simulink model "EMPlanner_cs_old"  (R2020a)
settings: Solver=ode5  StartTime=0.0  StopTime=55  FixedStep=1/1000  RelTol=1e-3
PreLoadFcn:
  | mbxruntime.callbacks.PreLoadFcn(bdroot);
PostLoadFcn:
  | mbxruntime.callbacks.PostLoadFcn(bdroot);
InitFcn:
  | mbxruntime.callbacks.InitFcn(bdroot);
StartFcn:
  | mbxruntime.callbacks.StartFcn(bdroot);
StopFcn:
  | mbxruntime.callbacks.StopFcn(bdroot);
model workspace: external: MAT-File .\EMPlanner_cs_hws.mat (data not in the file)
values from neighbouring files (symbols this model uses):
  c_factor = 43.75    [emplanner_init.m]
  cf = -175016    [emplanner_init.m]
  cr = -130634    [emplanner_init.m]
  KD_PID_distance = 0.0    (= 0)    [emplanner_init.m]
  KD_PID_speed = 0    [emplanner_init.m]
  KI_PID_distance = 0.0    (= 0)    [emplanner_init.m]
  KI_PID_speed = 0    [emplanner_init.m]
  KP_PID_distance = 0.5    [emplanner_init.m]
  KP_PID_speed = 1.8    [emplanner_init.m]
  la = 1.265    [emplanner_init.m]
  lb = 2.947-1.265    (= 1.682)    [emplanner_init.m]
  LQR_K1 = k(:,1)'    [emplanner_init.m]
  LQR_K2 = k(:,2)'    [emplanner_init.m]
  LQR_K3 = k(:,3)'    [emplanner_init.m]
  LQR_K4 = k(:,4)'    [emplanner_init.m]
  m = 2020    [emplanner_init.m]
  path_x = [7.7742 8.77358225507 9.77170536558 10.7685522493 11.7641171228 12.7583983581 13.7513958557 14.7431100776 15.7335416918 16.7226914411 17.7105600952 18.6971484329 ... (551 elements, 551x1)]    [test_path.mat]
  path_y = [-207.8202 -207.82020006 -207.820200616 -207.820202023 -207.82020429 -207.820207237 -207.820210603 -207.820214131 -207.82021762 -207.820220941 -207.820224011 -207.820226778 ... (551 elements, 551x1)]    [test_path.mat]
  rack_displacement = [-39.14 , -37.2 , -35.29 , -33.43 , -31.6 , -29.81 , -28.06 , -26.34 , -24.66 ,      -23.01 , -21.38 , -19.79 , -18.23 , -16.69 , -15.18 , -13.7 , -12.23 , -10.8 , -9.38 , -7.98 ,     -6.61 , -5.25 , -3.91 , -2.59 , -1.29 , 0 , 1.27 , 2.54 , 3.78 , 5.02 , 6.24 , 7.46 , 8.66 ,      9.86 , 11.05 , 12.24 , 13.41 , 14.59 , 15.76 , 16.92 , 18.09 , 19.25 , 20.42 , 21.59 , 22.76 ,      23.93 , 25.11 , 26 ...(+26 chars)    [emplanner_init.m]
  right_wheel_ground = [-70 ,-67.2 , -64.4 , -61.6 , -58.8 , -56 , -53.2 , -50.4 , -47.6 , -44.8 , -42 ,      -39.2 , -36.4 , -33.6 , -30.8 , -28 , -25.2 , -22.4 , -19.6 , -16.8 , -14 , -11.2 , -8.4 , -5.6 ,      -2.8 , 0 , 2.8 , 5.6 , 8.4 , 11.2 , 14 , 16.8 , 19.6 , 22.4 , 25.2 , 28 , 30.8 , 33.6 , 36.4 ,      39.2 , 42 , 44.8 , 47.6 , 50.4 , 53.2 , 56 , 58.8 , 61.6 , 64.4 , 67.2 , 70 ]    [emplanner_init.m]
  vx_break_point = zeros(1,5000)    [emplanner_init.m]
undefined symbols (not defined in the file or in its folder): aubr, DiscIntNeverNeededParam, tablebr, vubr, warningInitialVelocity, x0
libraries: simulink x19, PreScanSimulinkLibrary x10, simulink_extras x5, Solver_SF x1
(part 8 of 8)

== matlab function EMPlanner_cs_old/Audi_A8_Sedan_1/decision&planning module/EM Planner/Frenet2Cartesian ==
  data: s_set_fcs input; x_set_gcs output; l_set_fcs input; dl_set_fcs input; ddl_set_fcs input; path_x_set_gcs input; path_y_set_gcs input; path_heading_set_gcs input; path_kappa_set_gcs input; matchPoint_index_s_set_fcs input; y_set_gcs output; heading_set_gcs output; kappa_set_gcs output
function [x_set_gcs,y_set_gcs,heading_set_gcs,kappa_set_gcs] = fcn(s_set_fcs,l_set_fcs,dl_set_fcs,ddl_set_fcs,...
    path_x_set_gcs,path_y_set_gcs,path_heading_set_gcs,path_kappa_set_gcs,matchPoint_index_s_set_fcs)
% 该函数将批量将(s,l) 转化成 (x,y)
% s_set_fcs,l_set_fcs,dl_set_fcs,ddl_set_fcs 转换点 自然坐标系信息
% path_x_set_gcs,path_y_set_gcs,path_heading_set_gcs,path_kappa_set_gcs 给定路径采样点信息
% matchPoint_index_s_set_fcs 给定路径采样点s坐标集合
% 假设最多有181个点需要转换
n = 181;
% 输出初始化
x_set_gcs = ones(n,1)*nan; y_set_gcs = ones(n,1)*nan; heading_set_gcs = ones(n,1)*nan; kappa_set_gcs = ones(n,1)*nan;
for i = 1:length(s_set_fcs)
    if isnan(s_set_fcs(i))
        break;
    end
    % 求出该点在给定路径采样点上 投影点的信息
    [proj_point_x_gcs,proj_point_y_gcs,proj_point_heading_gcs,proj_point_kappa_gcs] = ...
                CalProjPointInfoFromFrenet(s_set_fcs(i),path_x_set_gcs,path_y_set_gcs,path_heading_set_gcs,...
                                                path_kappa_set_gcs,matchPoint_index_s_set_fcs);
    x_set_gcs(i) = proj_point_x_gcs - l_set_fcs(i) * sin(proj_point_heading_gcs);
    y_set_gcs(i) = proj_point_y_gcs + l_set_fcs(i) * cos(proj_point_heading_gcs);
    heading_set_gcs(i) = proj_point_heading_gcs + atan(dl_set_fcs(i)/(1-proj_point_kappa_gcs*l_set_fcs(i)));
    k1 = ddl_set_fcs(i) + proj_point_kappa_gcs * dl_set_fcs(i) * tan(heading_set_gcs(i)-proj_point_heading_gcs);
    k2 = (cos(heading_set_gcs(i)-proj_point_heading_gcs))^2 / (1 - proj_point_kappa_gcs*l_set_fcs(i));
    k3 = cos(heading_set_gcs(i)-proj_point_heading_gcs) / (1 - proj_point_kappa_gcs*l_set_fcs(i));
    kappa_set_gcs(i) = (k1 * k2 + proj_point_kappa_gcs) * k3;
end
end

== matlab function EMPlanner_cs_old/Audi_A8_Sedan_1/decision&planning module/EM Planner/path and speed merge ==
  data: s input; trajectory_x output; s_dot input; s_dot2 input; relative_time input; current_time input; path_s input; trajectory_x_init input; trajectory_y_init input; trajectory_heading_init input; trajectory_kappa_init input; trajectory_y output; trajectory_heading output; trajectory_kappa output; trajectory_speed output; trajectory_accel output; trajectory_time output
function [trajectory_x,trajectory_y,trajectory_heading,trajectory_kappa,trajectory_speed,trajectory_accel,trajectory_time] = ...
    fcn(s,s_dot,s_dot2,relative_time,current_time,path_s,trajectory_x_init,trajectory_y_init,trajectory_heading_init,trajectory_kappa_init)
% 该函数将合并path和speed
% 由于path 是 60个点，speed 有 401个点，合并后，path和speed有401个点，因此需要做插值
n = 401;
trajectory_x = zeros(n,1);
trajectory_y = zeros(n,1);
trajectory_heading = zeros(n,1);
trajectory_kappa = zeros(n,1);
trajectory_speed = zeros(n,1);

trajectory_accel = zeros(n,1);
index = 1;
% 由于trajectory_x_init中不是所有的值都有效，(有nan) 所以要找到有效值的范围
while ~isnan(trajectory_x_init(index)) 
    index = index + 1;
end
index = index - 1;
trajectory_time = zeros(n,1);
for i = 1:length(trajectory_heading_init)-1
    trajectory_heading_init(i+1) = trajectory_heading_init(i) + sin(trajectory_heading_init(i+1)-trajectory_heading_init(i));
end
for i = 1:n-1
    %interp1 线性插值
    % 若 x = [1,2] y = [3,4]
    %interp1(x,y,1.5) 会得到3.5
    %interp1 的缺点是 在端点或超过端点的，结果为nan
    % interp1(x,y,2) 不会等于4 而是会等于nan
    % interp1(x,y,6) 也会等于nan，所以在端点处要单独处理
    trajectory_x(i) = interp1(path_s(1:index),trajectory_x_init(1:index),s(i));
    trajectory_y(i) = interp1(path_s(1:index),trajectory_y_init(1:index),s(i));
    trajectory_heading(i) = interp1(path_s(1:index),trajectory_heading_init(1:index),s(i));
    trajectory_kappa(i) = interp1(path_s(1:index),trajectory_kappa_init(1:index),s(i));
    trajectory_time(i) = relative_time(i) + current_time;%速度规划会得到相对时间，转换成绝对时间
    trajectory_speed(i) = s_dot(i);
    trajectory_accel(i) = s_dot2(i);
end
% 端点单独处理
trajectory_x(end) = trajectory_x_init(end);
trajectory_y(end) = trajectory_y_init(end);
trajectory_heading(end) = trajectory_heading_init(end);
trajectory_kappa(end) = trajectory_kappa_init(end);
trajectory_time(end) = relative_time(end) + current_time;
trajectory_speed(end) = s_dot(end);
trajectory_accel(end) = s_dot2(end);

== matlab function EMPlanner_cs_old/Audi_A8_Sedan_1/decision&planning module/EM Planner/increase st point count ==
  data: s_init input; s output; s_dot_init input; s_dot2_init input; relative_time_init input; s_dot output; s_dot2 output; relative_time output
function [s,s_dot,s_dot2,relative_time] = fcn(s_init,s_dot_init,s_dot2_init,relative_time_init)
%该函数将增密s s_dot s_dot2
% 为什么需要增密，因为控制的执行频率是规划的10倍，轨迹点如果不够密，必然会导致规划效果不好
% 但是若在速度二次规划中点取的太多，会导致二次规划的矩阵规模太大计算太慢
% 所以方法是在二次规划中选取少量的点优化完毕后，在用此函数增密
T = relative_time_init(end);
n = 401;
dt = T/(n-1);
s = zeros(n,1);
s_dot = zeros(n,1);
s_dot2 = zeros(n,1);
relative_time = zeros(n,1);
for i = 1:n
    current_t = (i-1)*dt;
    for j = 1:length(relative_time_init)-1
        if relative_time_init(j) <= current_t && relative_time_init(j+1) > current_t
            break;
        end
    end
    x = current_t - relative_time_init(j);
    s(i) = s_init(j) + s_dot_init(j)*x + (1/3)*s_dot2_init(j)*x^2 + (1/6)*s_dot2_init(j+1)*x^2; 
    s_dot(i) = s_dot_init(j) + 0.5*s_dot2_init(j)*x + 0.5*s_dot2_init(j+1)*x;
    s_dot2(i) = s_dot2_init(j) + (s_dot2_init(j+1) - s_dot2_init(j))*x/(relative_time_init(j+1) - relative_time_init(j));
    relative_time(i) = current_t;
end

== matlab function EMPlanner_cs_old/Audi_A8_Sedan_1/decision&planning module/EM Planner/stitch trajectory ==
  data: trajectory_x input; trajectory_x_final output; trajectory_y input; trajectory_heading input; trajectory_kappa input; trajectory_speed input; trajectory_accel input; trajectory_time input; stitch_x input; stitch_y input; stitch_heading input; stitch_kappa input; stitch_speed input; stitch_accel input; stitch_time input; trajectory_y_final output; trajectory_heading_final output; trajectory_kappa_final output; trajectory_speed_final output; trajectory_accel_final output; trajectory_time_final output
function [trajectory_x_final,trajectory_y_final,trajectory_heading_final,trajectory_kappa_final,...
          trajectory_speed_final,trajectory_accel_final,trajectory_time_final] = fcn(trajectory_x,...
          trajectory_y,trajectory_heading,trajectory_kappa,trajectory_speed,trajectory_accel,trajectory_time,...
          stitch_x,stitch_y,stitch_heading,stitch_kappa,stitch_speed,stitch_accel,stitch_time)
% 轨迹拼接，把stitch trajectory 拼到规划完成的轨迹上
n = 401 + 20;
trajectory_x_final = zeros(n,1);
trajectory_y_final = zeros(n,1);
trajectory_heading_final = zeros(n,1);
trajectory_kappa_final = zeros(n,1);
trajectory_speed_final = zeros(n,1);
trajectory_accel_final = zeros(n,1);
trajectory_time_final = zeros(n,1);

trajectory_x_final = [stitch_x;trajectory_x];
trajectory_y_final = [stitch_y;trajectory_y];
trajectory_heading_final = [stitch_heading;trajectory_heading];
trajectory_kappa_final = [stitch_kappa;trajectory_kappa];
trajectory_speed_final = [stitch_speed;trajectory_speed];
trajectory_accel_final = [stitch_accel;trajectory_accel];
trajectory_time_final = [stitch_time;trajectory_time];

== matlab function EMPlanner_cs_old/Audi_A8_Sedan_1/decision&planning module/EM Planner/path decision with dynamic planning(dp) ==
  data: obs_s_set_fcs input; dpPath_s_init_set_fcs output; obs_l_set_fcs input; plan_startPoint_s_fcs input; plan_startPoint_l_fcs input; plan_startPoint_dl_fcs input; plan_startPoint_ddl_fcs input; w_obs input; w_smooth_dl input; w_smooth_ddl input; w_smooth_dddl input; w_ref input; row input; col input; sample_s input; sample_l input; dpPath_l_init_set_fcs output
function [dpPath_s_init_set_fcs,dpPath_l_init_set_fcs] = fcn(obs_s_set_fcs,obs_l_set_fcs,plan_startPoint_s_fcs,...
    plan_startPoint_l_fcs,plan_startPoint_dl_fcs,plan_startPoint_ddl_fcs,...
         w_obs,w_smooth_dl,w_smooth_ddl,w_smooth_dddl,w_ref,row,col,sample_s,sample_l)
% 该函数将通过动态规划出一条初始路径来实现避障
% obs_s_set_fcs,obs_l_set_fcs 障碍物坐标信息
% plan_startPoint_s_fcs,plan_startPoint_l_fcs,plan_startPoint_dl_fcs,plan_startPoint_ddl_fcs 规划起点信息
%  w_obs,w_smooth_dl,w_smooth_ddl,w_smooth_dddl,w_ref 动态规划权重参数
% 采样点的行 列 行间距 列间距  行数必须为技术  且中间行的点需要刚好在s轴上
mid_row = (row+1)/2;
% dpPath_s_init_set_fcs,dpPath_l_init_set_fcs  暂时不包括规划起点
% 输出初始化
% 假设最多取20列采样点
max_col = 20;
dpPath_s_init_set_fcs = ones(max_col,1) * nan; dpPath_l_init_set_fcs = ones(max_col,1) * nan;
node_minCost_set = ones(row,col) * inf; % 用来记录自车从规划起点到每个采样点的最小代价
preCol_bestRow_set = zeros(row, col); % 用来记录到达该采样点最优路径前一列的行号   第一列采样点前一列最优行号视为0

% 首先计算规划起点到第一列所有采样点的代价
for i = 1:row
    pre_col_node_s_fcs = plan_startPoint_s_fcs; pre_col_node_l_fcs = plan_startPoint_l_fcs;
    pre_col_node_dl_fcs = plan_startPoint_dl_fcs; pre_col_node_ddl_fcs = plan_startPoint_ddl_fcs;
    cur_col_node_s_fcs = plan_startPoint_s_fcs + sample_s;
    cur_col_node_l_fcs = (mid_row - i) * sample_l;
    cur_col_node_dl_fcs = 0; cur_col_node_ddl_fcs = 0;
    node_minCost_set(i,1) = CalNeighbourColPointCost(pre_col_node_s_fcs,pre_col_node_l_fcs,pre_col_node_dl_fcs,pre_col_node_ddl_fcs,...
    cur_col_node_s_fcs, cur_col_node_l_fcs,cur_col_node_dl_fcs,cur_col_node_ddl_fcs, w_obs,w_smooth_dl,w_smooth_ddl,...
    w_smooth_dddl,w_ref,obs_s_set_fcs,obs_l_set_fcs,sample_s);
end

% 再计算规划起点到后续列所有采样点的最小代价 以及最优轨迹行数
% 一列一列的往后遍历
for j = 2:col
    for i = 1:row
        %遍历当前列所有行
        cur_col = j;
        cur_col_node_s_fcs = plan_startPoint_s_fcs + cur_col * sample_s;
        cur_col_node_l_fcs = (mid_row - i) * sample_l;
        cur_col_node_dl_fcs = 0; cur_col_node_ddl_fcs = 0;
        % 求解前一列所有行采样点到当前列当前行采样点的代价
        for k = 1:row
            % 遍历前一列所有行
            pre_col = j - 1;
            pre_col_node_s_fcs = plan_startPoint_s_fcs + pre_col * sample_s;
            pre_col_node_l_fcs = (mid_row - k) * sample_l;
            pre_col_node_dl_fcs = 0; pre_col_node_ddl_fcs = 0;
            % 前一列当前行采样点到当前列当前行采样点的代价
            cost = CalNeighbourColPointCost(pre_col_node_s_fcs,pre_col_node_l_fcs,pre_col_node_dl_fcs,pre_col_node_ddl_fcs,...
                cur_col_node_s_fcs, cur_col_node_l_fcs,cur_col_node_dl_fcs,cur_col_node_ddl_fcs, w_obs,w_smooth_dl,w_smooth_ddl,...
                w_smooth_dddl,w_ref,obs_s_set_fcs,obs_l_set_fcs,sample_s);
            cost = cost + node_minCost_set(k,pre_col);
            % 通过比较 最终将最小代价填充进数组
            if cost < node_minCost_set(i,cur_col)
                node_minCost_set(i,cur_col) = cost;
                preCol_bestRow_set(i,cur_col) = k;
            end
        end
    end
end

% 计算最后一列最优路径点是哪个  亦即是最终目标点
% 即计算数组node_minCost_set最后一列对应行数
lastCol_bestRow = 0;
minCost = inf;
for i = 1:row
    if node_minCost_set(i,end) < minCost
        lastCol_bestRow = i;
        minCost = node_minCost_set(i,end);
    end
end
best_row_set = zeros(col,1); best_row_set(end) = lastCol_bestRow;
best_row = lastCol_bestRow;
% 再计算到达最后一列最优路径点 前面所经历过的轨迹行数
for j = col:-1:2
    best_row = preCol_bestRow_set(best_row,j);
    best_row_set(j-1) = best_row;
end

% 根据最优路径行号 求解最优路径采样点坐标
for j = 1:col
    if j > max_col
        break;
    end
    dpPath_s_init_set_fcs(j) = plan_startPoint_s_fcs + j * sample_s;
    dpPath_l_init_set_fcs(j) = (mid_row - best_row_set(j)) * sample_l;
end
end

== matlab function EMPlanner_cs_old/Audi_A8_Sedan_1/decision&planning module/referenceline provider/MATLAB Function1 ==
  data: x_set_gcs input; match_point_index_set output; y_set_gcs input; path_x_set_gcs input; path_y_set_gcs input; path_heading_set_gcs input; path_kappa_set_gcs input; proj_point_x_set_gcs output; proj_point_y_set_gcs output; proj_point_heading_set_gcs output; proj_point_kappa_set_gcs output
function [match_point_index_set,proj_point_x_set_gcs,proj_point_y_set_gcs,proj_point_heading_set_gcs,...
    proj_point_kappa_set_gcs] = fcn(x_set_gcs,y_set_gcs,path_x_set_gcs,path_y_set_gcs,...
    path_heading_set_gcs,path_kappa_set_gcs)
% 该函数将批量计算点在给定路径下的匹配点编号和投影点信息   
% x_set_gcs,y_set_gcs 输入点信息集合
% path_x_set_gcs,path_y_set_gcs,path_heading_set_gcs,path_kappa_set_gcs 给定路径点信息集合
% match_point_index_set 匹配点编号集合
% proj_point_x_set_gcs,proj_point_y_set_gcs,proj_point_heading_set_gcs,proj_point_kappa_set_gcs 投影点信息集合

% 假设最多有181个点需要投影
n = 181;
% 对输出进行初始化
match_point_index_set = ones(n,1) *nan; 
proj_point_x_set_gcs = ones(n,1) *nan;  proj_point_y_set_gcs = ones(n,1) *nan;
proj_point_heading_set_gcs = ones(n,1) *nan;  proj_point_kappa_set_gcs = ones(n,1) *nan;

% 寻找匹配点时 需要利用上一个周期的结果 因此定义需要利用的静态变量
persistent is_first_run;
persistent pre_match_point_index_set;
persistent pre_path_x_set_gcs; persistent pre_path_y_set_gcs; % 通过上个周期匹配点位矢判断遍历方向
persistent pre_path_heading_set_gcs; persistent pre_path_kappa_set_gcs;
persistent pre_x_set_gcs; persistent pre_y_set_gcs; % 判断相邻帧检测的是否是同一个障碍物

if isempty(is_first_run)
    is_first_run = 0;
    % 首次运行 所有待求点都从给定路径路径第一个点开始找 往前遍历 且距离连续增长上限设为50
    for i = 1:length(x_set_gcs) % 存在的点都在前面 遍历到nan至后面的点都不存在
        if isnan(x_set_gcs(i))
            break;
        end
        start_find_index = 1; forward_stable_backward = 1; increase_count_limit = 50;
        % 计算匹配点编号
        match_point_index = CalMatchPointIndex(x_set_gcs(i),y_set_gcs(i),path_x_set_gcs,...
        path_y_set_gcs,path_heading_set_gcs,path_kappa_set_gcs,start_find_index,...
        increase_count_limit, forward_stable_backward);
        % 计算投影点信息
        [proj_point_x_gcs,proj_point_y_gcs,proj_point_heading_gcs,proj_point_kappa_gcs] = ...
        CalProjPointInfo(x_set_gcs(i),y_set_gcs(i),path_x_set_gcs,path_y_set_gcs,path_heading_set_gcs,...
        path_kappa_set_gcs,match_point_index);
        % 将每个点求解信息添加到集合
        match_point_index_set(i) = match_point_index;
        proj_point_x_set_gcs(i) = proj_point_x_gcs; proj_point_y_set_gcs(i) = proj_point_y_gcs;
        proj_point_heading_set_gcs(i) = proj_point_heading_gcs; 
        proj_point_kappa_set_gcs(i) = proj_point_kappa_gcs;
    end
    % 保存该周期信息 以便下周期使用
    pre_match_point_index_set = match_point_index_set;
    pre_path_x_set_gcs = path_x_set_gcs; pre_path_y_set_gcs = path_y_set_gcs;
    pre_path_heading_set_gcs = path_heading_set_gcs; pre_path_kappa_set_gcs = path_kappa_set_gcs;
    pre_x_set_gcs = x_set_gcs; pre_y_set_gcs = y_set_gcs;
else
    % 需要使用上周期信息
    for i = 1:length(x_set_gcs)
        if isnan(x_set_gcs(i))
            break;
        end
        % 检测相邻帧是否是同一物体求解
        dis = sqrt((x_set_gcs(i)-pre_x_set_gcs(i))^2 + (y_set_gcs(i)-pre_y_set_gcs(i))^2);
        if dis > 10  % 相邻帧(相隔0.1s)同一物体距离不可能这么大
            % 说明相邻帧不是同一物体 上周期该物体已经消失在车辆的检测范围内
            % 把上周期该物体匹配点编号信息清空
            pre_match_point_index_set(i) = nan;
        end
        if isnan(pre_match_point_index_set(i))
            % 说明该物体是第一次寻找匹配点 从头开始寻找 且往前遍历
            start_find_index = 1; forward_stable_backward = 1; increase_count_limit = 50;
        else
            % 说明该物体上周期已经寻找过匹配点  判断开始寻找编号 和遍历方向
            start_find_index = pre_match_point_index_set(i); increase_count_limit = 5;
            % 提取上周期匹配点信息
            pre_match_point_x = pre_path_x_set_gcs(pre_match_point_index_set(i));
            pre_match_point_y = pre_path_y_set_gcs(pre_match_point_index_set(i));
            pre_match_point_heading = pre_path_heading_set_gcs(pre_match_point_index_set(i));
            % 通过该物体上周期匹配点位置到本周期位置向量和上周期匹配点切向量的点乘来判断遍历方向
            vector_preMatch_current = [x_set_gcs(i),y_set_gcs(i)] - [pre_match_point_x, pre_match_point_y];
            vector_tor_preMatch = [cos(pre_match_point_heading), sin(pre_match_point_heading)];
            forward_stable_backward = dot(vector_preMatch_current, vector_tor_preMatch);
        end
        % 计算匹配点编号
        match_point_index = CalMatchPointIndex(x_set_gcs(i),y_set_gcs(i),path_x_set_gcs,...
        path_y_set_gcs,path_heading_set_gcs,path_kappa_set_gcs,start_find_index,...
        increase_count_limit, forward_stable_backward);
        % 计算投影点信息
        [proj_point_x_gcs,proj_point_y_gcs,proj_point_heading_gcs,proj_point_kappa_gcs] = ...
        CalProjPointInfo(x_set_gcs(i),y_set_gcs(i),path_x_set_gcs,path_y_set_gcs,path_heading_set_gcs,...
        path_kappa_set_gcs,match_point_index);
        % 将每个点求解信息添加到集合
        match_point_index_set(i) = match_point_index;
        proj_point_x_set_gcs(i) = proj_point_x_gcs; proj_point_y_set_gcs(i) = proj_point_y_gcs;
        proj_point_heading_set_gcs(i) = proj_point_heading_gcs; 
        proj_point_kappa_set_gcs(i) = proj_point_kappa_gcs;
    end
    % 保存该周期信息 以便下周期使用
    pre_match_point_index_set = match_point_index_set;
    pre_path_x_set_gcs = path_x_set_gcs; pre_path_y_set_gcs = path_y_set_gcs;
    pre_path_heading_set_gcs = path_heading_set_gcs; pre_path_kappa_set_gcs = path_kappa_set_gcs;
    pre_x_set_gcs = x_set_gcs; pre_y_set_gcs = y_set_gcs;
end
end

== matlab function EMPlanner_cs_old/Audi_A8_Sedan_1/control module2/control main/lateral control LQR/calc lqr K ==
  data: k1 input; k output; k2 input; k3 input; k4 input; vx input
function k  = fcn(k1,k2,k3,k4,vx)
    if abs(vx)<0.1
        k=[0,0,0,0];
    else
       
        k=[k1,k2,k3,k4];
    end
end

== matlab function EMPlanner_cs_old/Audi_A8_Sedan_1/control module2/control main/lateral control LQR/err_kappa_calculate_module ==
  data: x input; y input; phi input; vx input; vy input; phi_dot input; xr input; yr input; thetar input; kappar input; err output; es output; s_dot output; phi output; projection_point_thetar output
function [err,es,s_dot,phi,projection_point_thetar] = fcn(x,y,phi,vx,vy,phi_dot,xr,yr,thetar,kappar)
    
    tor=[cos(thetar);sin(thetar)];
    nor=[-sin(thetar);cos(thetar)];
    d_err=[x-xr;y-yr];
    ed=nor'*d_err;
    es=tor'*d_err;
    %projection_point_thetar=thetar(dmin);%apollo
    projection_point_thetar=thetar+kappar*es;
    ed_dot=vy*cos(phi-projection_point_thetar)+vx*sin(phi-projection_point_thetar);
    %%%%%%%%%
    ephi=sin(phi-projection_point_thetar);
    %%%%%%%%%
    ss_dot=vx*cos(phi-projection_point_thetar)-vy*sin(phi-projection_point_thetar);
    s_dot=ss_dot/(1-kappar*ed);
    ephi_dot=phi_dot-kappar*s_dot;
    err=[ed;ed_dot;ephi;ephi_dot];
    
    
    
    
    
    
    
    
    
    
    
    


end

== matlab function EMPlanner_cs_old/Audi_A8_Sedan_1/control module2/control main/lateral control LQR/feed_forword_control ==
  data: vx input; a input; forword_angle output; b input; m input; cf input; cr input; k input; kr input
function forword_angle = fcn(vx,a,b,m,cf,cr,k,kr)
    forword_angle=kr*(a+b-b*k(3)-(m*vx*vx/(a+b))*((b/cf)+(a/cr)*k(3)-(a/cr)));
end

== matlab function EMPlanner_cs_old/Audi_A8_Sedan_1/control module2/control main/lateral control LQR/feedback_control+feedforword_control ==
  data: k input; angle output; err input; forword_angle input
function angle = fcn(k,err,forword_angle)

    angle=-k*err+forword_angle;
end

== matlab function EMPlanner_cs_old/Audi_A8_Sedan_1/control module2/control main/lateral control LQR/predict_module ==
  data: x input; pred_x_ctrl output; y input; phi input; vx input; vy input; phi_dot input; ts input; pred_y_ctrl output; pred_yaw_ctrl output; pred_vx_ctrl output; pred_vy_ctrl output; pred_yaw_dot_ctrl output
function [pred_x_ctrl,pred_y_ctrl,pred_yaw_ctrl,pred_vx_ctrl,pred_vy_ctrl,pred_yaw_dot_ctrl] = fcn(x,y,phi,vx,vy,phi_dot,ts)
    pred_x_ctrl=x+vx*ts*cos(phi)-vy*ts*sin(phi);
    pred_y_ctrl=y+vy*ts*cos(phi)+vx*ts*sin(phi);
    pred_yaw_ctrl=phi;
    pred_vx_ctrl=vx;
    pred_vy_ctrl=vy;
    pred_yaw_dot_ctrl=phi_dot;
end

== matlab function EMPlanner_cs_old/Audi_A8_Sedan_1/control module2/control main/longitudinal control double PID/MATLAB Function1 ==
  data: u input; throttle output; brake output
function [throttle,brake] = fcn(u)
    if u>=0
        throttle=u;
        brake=0;
    else
        throttle=0;
        brake=-u;
    end

== matlab function EMPlanner_cs_old/Audi_A8_Sedan_1/decision&planning module/EM Planner/calc speed planning start condition ==
  data: plan_start_vx input; plan_start_s_dot output; plan_start_vy input; plan_start_ax input; plan_start_ay input; plan_start_heading input; plan_start_s_dot2 output
function [plan_start_s_dot,plan_start_s_dot2] = fcn(plan_start_vx,plan_start_vy,plan_start_ax,plan_start_ay,plan_start_heading)
% 该函数计算速度规划的初始条件
tor = [cos(plan_start_heading);sin(plan_start_heading)];
v_t = tor'*[plan_start_vx;plan_start_vy];
a_t = tor'*[plan_start_ax;plan_start_ay];
plan_start_s_dot = v_t;
plan_start_s_dot2 = a_t;

== matlab function EMPlanner_cs_old/Audi_A8_Sedan_1/decision&planning module/EM Planner/simple speed qp planning ==
  data: plan_start_s_dot input; s_init output; plan_start_s_dot2 input; s_end input; recommend_T input; s_dot_init output; s_dot2_init output; relative_time_init output
function [s_init,s_dot_init,s_dot2_init,relative_time_init] = fcn(plan_start_s_dot,plan_start_s_dot2,s_end,recommend_T)
%简单速度二次规划
coder.extrinsic("quadprog")
n = 51;
s_init = zeros(n,1);
s_dot_init = zeros(n,1);
s_dot2_init = zeros(n,1);
relative_time_init = zeros(n,1);

Aeq = zeros(3*n,2*n - 2);
beq = zeros(2*n - 2,1);
lb = ones(3*n,1);
ub = lb;
dt = recommend_T/(n-1);
A_sub =[1,0;
        dt,1;
        (1/3)*dt^2,(1/2)*dt;
        -1,0;
        0,-1;
        (1/6)*dt^2,dt/2];
for i = 1:n - 1
    Aeq(3*i-2:3*i+3,2*i-1:2*i) = A_sub;
end

for i = 1:n
   lb(3*i - 2) = -inf;
   lb(3*i - 1) = 0;
   lb(3*i) = -8;
   ub(3*i - 2) = inf;
   ub(3*i - 1) = 50;
   ub(3*i) = 2;
end
lb(1) = 0;
lb(2) = plan_start_s_dot;
lb(3) = plan_start_s_dot2;
ub(1) = lb(1);
ub(2) = lb(2);
ub(3) = lb(3);
lb(3*n - 2) = s_end;
ub(3*n - 2) = s_end;
A3 = zeros(3*n,3*n);
A4 = zeros(3*n,n - 1);
A4_sub =[0;0;1;0;0;-1];
for i = 1:n - 1
   A3(3*i,3*i) = 1;
   A4(3*i-2:3*i+3,i:i) = A4_sub;
end
A3(3*n,3*n) = 1;
H = A3 + 100*(A4*A4');
H = 2*H;
f = zeros(3*n,1);
X = quadprog(H,f,[],[],Aeq',beq,lb,ub);
for i = 1:n
   s_init(i) = X(3*i - 2);
   s_dot_init(i) = X(3*i - 1);
   s_dot2_init(i) = X(3*i);
   relative_time_init(i) = (i - 1)*dt;
end

== matlab function EMPlanner_cs_old/Audi_A8_Sedan_1/perception module 自车感知模块/计算出障碍物的绝对位置信息和速度信息 ==
  data: host_x_gcs input; obs_x_set_gcs output; host_y_gcs input; host_heading_gcs input; obs_range_set_sensor input; obs_y_set_gcs output; obs_velocity_set_gcs output; obs_velocity_heading_set_gcs output; obs_theta_set_sensor input; obs_velocity_set_sensor input; obs_velocity_heading_set_sensor input
function [obs_x_set_gcs,obs_y_set_gcs,obs_velocity_set_gcs,obs_velocity_heading_set_gcs] = ...
    fcn(host_x_gcs,host_y_gcs,host_heading_gcs,obs_range_set_sensor,obs_theta_set_sensor,obs_velocity_set_sensor,obs_velocity_heading_set_sensor)
% gcs 全局坐标系   global coordinate system
% 感知模块
% 输入：host_x,host_y,host_heading 自身车辆信息
% obs_range_set_sensor,obs_theta_set_sensor,obs_velocity_set_sensor,obs_velocity_heading_set_sensor 传感器检测到的障碍物信息
% range:障碍物离传感器的直线距离
% theta: 车辆前进方向与障碍物和传感器连线的夹角 顺时针为正 逆时针为负
% velocity:传感器检测到的障碍物的绝对速度
% velocity_heading:障碍物的速度与正北方向的夹角 以北为轴 顺时针旋转为正
% 输出:obs_x_set_gcs,obs_y_set_gcs,obs_velocity_set_gcs,obs_velocity_heading_set_gcs 障碍物在全局坐标下的信息
% 传感器最多识别n个障碍物   n是固定的  即为传感器最多检测障碍物的个数
% 输出初始化
n = length(obs_range_set_sensor);
obs_x_set_gcs = ones(n, 1) * nan;
obs_y_set_gcs = ones(n, 1) * nan;
obs_velocity_set_gcs = ones(n, 1) * nan;
obs_velocity_heading_set_gcs = ones(n, 1) * nan;
% for i = 1:n
%     % 把当前检测到的障碍物信息放进数组 没有检测到的置为nan 
%     % 相当于当前检测到的障碍物都放在数组前面  等到nan为止表示后面的障碍物都不存在
%     if  obs_range_set_sensor(i) ~= 0  %等于0时表示传感器没有检测到该障碍物  无需计算 或者该障碍物不存在
%         % 相邻帧之间障碍物的下标不会改变
%         % 2.16 为传感器到车辆质心的距离
%         obs_x_set_gcs(count) = host_x_gcs + 2.16*cos(host_heading_gcs) + obs_range_set_sensor(i)*cos(host_heading_gcs-obs_theta_set_sensor(i));
%         obs_y_set_gcs(count) = host_y_gcs + 2.16*sin(host_heading_gcs) + obs_range_set_sensor(i)*sin(host_heading_gcs-obs_theta_set_sensor(i));
%         obs_velocity_set_gcs(count) = obs_velocity_set_sensor(i);
%         obs_velocity_heading_set_gcs(count) = pi/2 - obs_velocity_heading_set_sensor(i);
%         count = count + 1;
%     end
% end
for i = 1:n
    % 把当前检测到的障碍物信息放进数组 没有检测到的置为nan 
    % 相当于当前检测到的障碍物都放在数组前面  等到nan为止表示后面的障碍物都不存在
    if  obs_range_set_sensor(i) ~= 0  %等于0时表示传感器没有检测到该障碍物  无需计算 或者该障碍物不存在
        % 相邻帧之间障碍物的下标不会改变
        % 2.16 为传感器到车辆质心的距离
        obs_x_set_gcs(i) = host_x_gcs + 2.16*cos(host_heading_gcs) + obs_range_set_sensor(i)*cos(host_heading_gcs-obs_theta_set_sensor(i));
        obs_y_set_gcs(i) = host_y_gcs + 2.16*sin(host_heading_gcs) + obs_range_set_sensor(i)*sin(host_heading_gcs-obs_theta_set_sensor(i));
        obs_velocity_set_gcs(i) = obs_velocity_set_sensor(i);
        obs_velocity_heading_set_gcs(i) = pi/2 - obs_velocity_heading_set_sensor(i);
    end
end

end

== matlab function EMPlanner_cs_old/Audi_A8_Sedan_1/decision&planning module/referenceline provider/MATLAB Function2 ==
  data: host_match_point_index input; referenceline_x_init_set_gcs output; path_x_set_gcs input; path_y_set_gcs input; referenceline_y_init_set_gcs output
function [referenceline_x_init_set_gcs, referenceline_y_init_set_gcs] = fun(host_match_point_index, ...
    path_x_set_gcs, path_y_set_gcs)
% 该函数将在给定路径上提取初始参考线
%  host_match_point_index 自车在给定路径上匹配点编号
%  path_x_set_gcs, path_y_set_gcs 给定路径坐标信息
%  referenceline_x_init_set_gcs, referenceline_y_init_set_gcs 初始参考线信息
% 在给定路径上 由匹配点编号往前进方向取150个点  往后退方向取30个点  总共181个点  给定路径一般肯定会多于181个点
% 需要判断 前进方向是否有150个点  或者后退方向是否有30个点
% 从起点着手  一定取得是181个点
if host_match_point_index <= 30
    % 后退方向不够30个点
    start_index = 1; % 从起点开始取
elseif host_match_point_index + 150 > length(path_x_set_gcs)
    % 前进方向不够150个点 则后退方向多取些点
    start_index = length(path_x_set_gcs) - 180;
else
    % 前进和后退方向点的数量均满足要求
    start_index = host_match_point_index - 30;
end

% 在给定路径上提取181个点作为初始参考线 
% referenceline_x_init_set_gcs = path_x_set_gcs(start_index:end_index); %不支持变矩阵
% referenceline_y_init_set_gcs = path_y_set_gcs(start_index:end_index);
referenceline_x_init_set_gcs = path_x_set_gcs(start_index:start_index + 180);
referenceline_y_init_set_gcs = path_y_set_gcs(start_index:start_index + 180);
end
